simulink model "fazova_trajektorie_2"  (R2018a)
settings: Solver=VariableStepAuto  StartTime=0.0  StopTime=100  RelTol=1e-3
undefined symbols (not defined in the file): w0
libraries: simulink x1
settings Model: Creator=vejvarm  LastModifiedBy=Martin

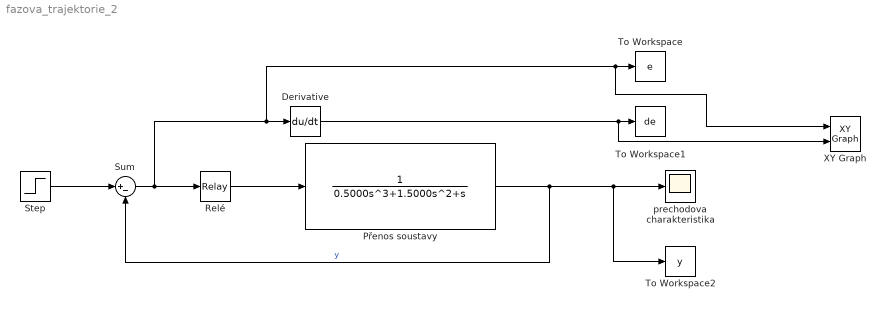
== system fazova_trajektorie_2 ==
  Derivative : Derivative
  Přenos soustavy : TransferFcn  Denominator=[0.5000 1.5000 1.0000 0]
  Relé : Relay  OnSwitchValue=0  OffSwitchValue=0  OnOutputValue=0.5  OffOutputValue=-0.5
  Step : Step  Time=0  After=w0  SampleTime=0
  Sum : Sum  Inputs=|+-
  To Workspace : ToWorkspace  VariableName=e  SaveFormat=Structure With Time  SampleTime=-1
  To Workspace1 : ToWorkspace  VariableName=de  SaveFormat=Structure With Time  SampleTime=-1
  To Workspace2 : ToWorkspace  VariableName=y  SaveFormat=Structure With Time  SampleTime=-1
  XY Graph : simulink/Sinks/XY Graph  xmin=-1  xmax=1  ymin=-1  ymax=1  st=-1
  prechodova charakteristika : Scope
  wires:
  Relé/1 -> Přenos soustavy/1
  Sum/1 -> Relé/1, XY Graph/1, To Workspace/1, Derivative/1
  Přenos soustavy/1 -> Sum/2, To Workspace2/1, prechodova charakteristika/1  "y"
  Derivative/1 -> XY Graph/2, To Workspace1/1
  Step/1 -> Sum/1
